simulink model "s2"  (R2019b)
settings: Solver=VariableStepAuto  StartTime=0.0  StopTime=10.0  RelTol=1e-3
values from neighbouring files (symbols this model uses):
  C = 10e-6    (= 1e-05)    [ex1.m]
  L = 1e-3    (= 0.001)    [ex1.m]
  R = 10    [ex1.m]
settings Model: Creator=Emanuel Pereira  LastModifiedBy=Emanuel Pereira

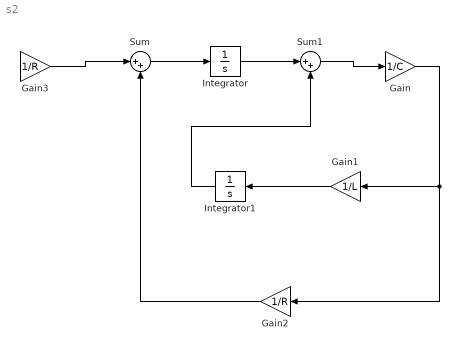
== system s2 ==
  Gain : Gain  Gain=1/C
  Gain1 : Gain  Gain=1/L
  Gain2 : Gain  Gain=1/R
  Gain3 : Gain  Gain=1/R
  Integrator : Integrator
  Integrator1 : Integrator
  Sum : Sum  Inputs=|++
  Sum1 : Sum  Inputs=|++
  wires:
  Sum/1 -> Integrator/1
  Integrator/1 -> Sum1/1
  Sum1/1 -> Gain/1
  Gain/1 -> Gain2/1, Gain1/1
  Gain1/1 -> Integrator1/1
  Integrator1/1 -> Sum1/2
  Gain2/1 -> Sum/2
  Gain3/1 -> Sum/1
